simulink model "PROBLEM_2_SUSPENSION_SYSTEM"  (R2020b)
settings: Solver=VariableStepAuto  StartTime=0.0  StopTime=10.0  RelTol=1e-3
undefined symbols (not defined in the file): a, b, c, d, den, num
settings Model: Creator=intel  LastModifiedBy=intel

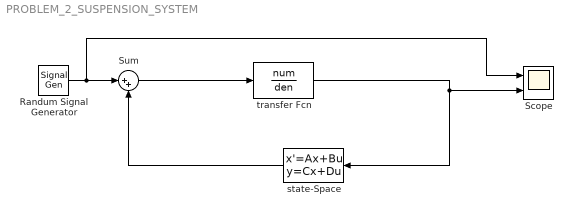
== system PROBLEM_2_SUSPENSION_SYSTEM ==
  Randum Signal Generator : SignalGenerator  WaveForm=random  Units=rad/sec
  Scope : Scope  NumInputPorts=2
  Sum : Sum  Inputs=|++
  state-Space : StateSpace  A=a  B=b  C=c  D=d  InitialCondition=0
  transfer Fcn : TransferFcn  Numerator=num  Denominator=den
  wires:
  Sum/1 -> transfer Fcn/1
  transfer Fcn/1 -> Scope/2, state-Space/1
  Randum Signal Generator/1 -> Scope/1, Sum/1
  state-Space/1 -> Sum/2
